simulink model "CP_ContrSys_Lin_b_n9945008"  (R2018b)
settings: Solver=VariableStepAuto  StartTime=0.0  StopTime=5  RelTol=1e-3
values from neighbouring files (symbols this model uses):
  Ab = [ 0 ,          0           , 1 , 0 ... (first row only)    [CP_ContrSys_Lin_b_MainFile_n9945008.m]
  Bb = [0;0;1/Mc;1/(l*Mc)]    [CP_ContrSys_Lin_b_MainFile_n9945008.m]
  Cb = [1,0,0,0 ... (first row only)    [CP_ContrSys_Lin_b_MainFile_n9945008.m]
  Kb = place(Ab, Bb, [-3,-4,-5,-6])    [CP_ContrSys_Lin_b_MainFile_n9945008.m]
  Lb = place(Ab',Cb', [-63,-64,-65,-66])'    [CP_ContrSys_Lin_b_MainFile_n9945008.m]
  x0 = [0.2 200*pi/180 0 0]'    [CP_ContrSys_Lin_b_MainFile_n9945008.m]
  xbar = [0;pi;0;0]    [CP_ContrSys_Lin_b_MainFile_n9945008.m]
settings Model: Creator=n9945008  LastModifiedBy=cody

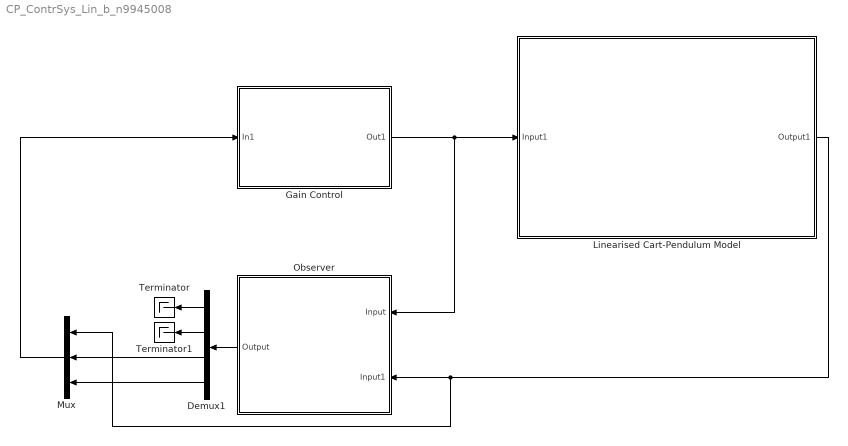
== system CP_ContrSys_Lin_b_n9945008 ==
  Demux1 : Demux
  Gain Control : Subsystem
  "Linearised Cart-Pendulum Model " : Subsystem
  Mux : Mux  Inputs=3
  Observer : Subsystem
  Terminator : Terminator
  Terminator1 : Terminator
  wires:
  Gain Control/1(Out1) -> "Linearised Cart-Pendulum Model "/1(Input1), Observer/1(Input)
  Observer/1(Output) -> Demux1/1
  Demux1/1 -> Terminator/1
  Demux1/2 -> Terminator1/1
  Demux1/3 -> Mux/2
  Demux1/4 -> Mux/3
  Mux/1 -> Gain Control/1(In1)
  "Linearised Cart-Pendulum Model "/1(Output1) -> Mux/1, Observer/2(Input1)

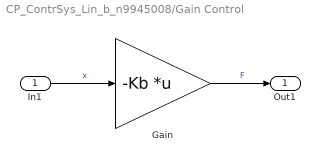
== system CP_ContrSys_Lin_b_n9945008/Gain Control ==
  In1 : Inport
  Gain : Gain  Gain=-Kb  Multiplication=Matrix(K*u)
  Out1 : Outport
  wires:
  In1/1 -> Gain/1  "x"
  Gain/1 -> Out1/1  "F"

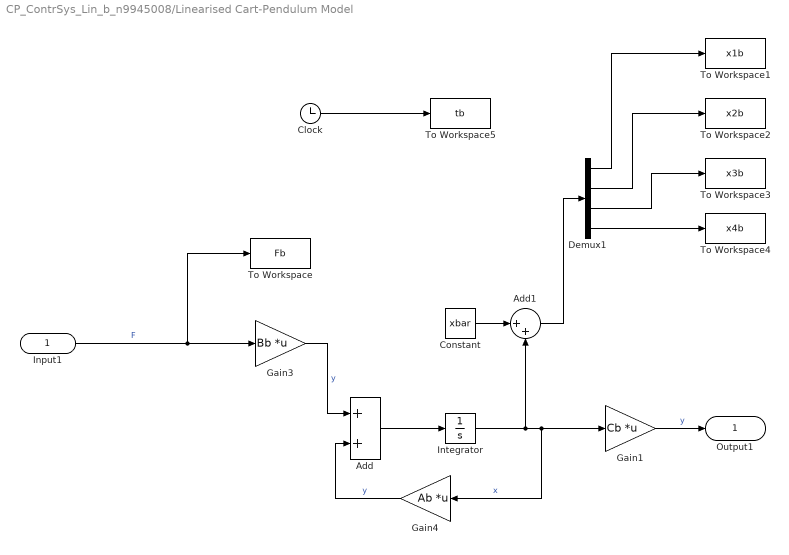
== system CP_ContrSys_Lin_b_n9945008/Linearised Cart-Pendulum Model  ==
  Input1 : Inport
  Add : Sum  Inputs=2
  Add1 : Sum  Inputs=|++
  Clock : Clock
  Constant : Constant  Value=xbar
  Demux1 : Demux
  Gain1 : Gain  Gain=Cb  Multiplication=Matrix(K*u)
  Gain3 : Gain  Gain=Bb  Multiplication=Matrix(K*u)
  Gain4 : Gain  Gain=Ab  Multiplication=Matrix(K*u)
  Integrator : Integrator  InitialCondition=x0-xbar
  To Workspace : ToWorkspace  VariableName=Fb  SampleTime=-1
      settings: Save2DSignal=2-D array (concatenate along first dimension)
  To Workspace1 : ToWorkspace  VariableName=x1b  SampleTime=-1
      settings: Save2DSignal=2-D array (concatenate along first dimension)
  To Workspace2 : ToWorkspace  VariableName=x2b  SampleTime=-1
      settings: Save2DSignal=2-D array (concatenate along first dimension)
  To Workspace3 : ToWorkspace  VariableName=x3b  SampleTime=-1
      settings: Save2DSignal=2-D array (concatenate along first dimension)
  To Workspace4 : ToWorkspace  VariableName=x4b  SampleTime=-1
      settings: Save2DSignal=2-D array (concatenate along first dimension)
  To Workspace5 : ToWorkspace  VariableName=tb  SampleTime=-1
      settings: Save2DSignal=2-D array (concatenate along first dimension)
  Output1 : Outport
  wires:
  Gain1/1 -> Output1/1  "y"
  Add/1 -> Integrator/1
  Demux1/3 -> To Workspace3/1
  Integrator/1 -> Gain1/1, Gain4/1, Add1/2  "x"
  Demux1/2 -> To Workspace2/1
  Clock/1 -> To Workspace5/1
  Gain3/1 -> Add/1  "y"
  Gain4/1 -> Add/2  "y"
  Demux1/4 -> To Workspace4/1
  Input1/1 -> To Workspace/1, Gain3/1  "F"
  Demux1/1 -> To Workspace1/1
  Constant/1 -> Add1/1
  Add1/1 -> Demux1/1

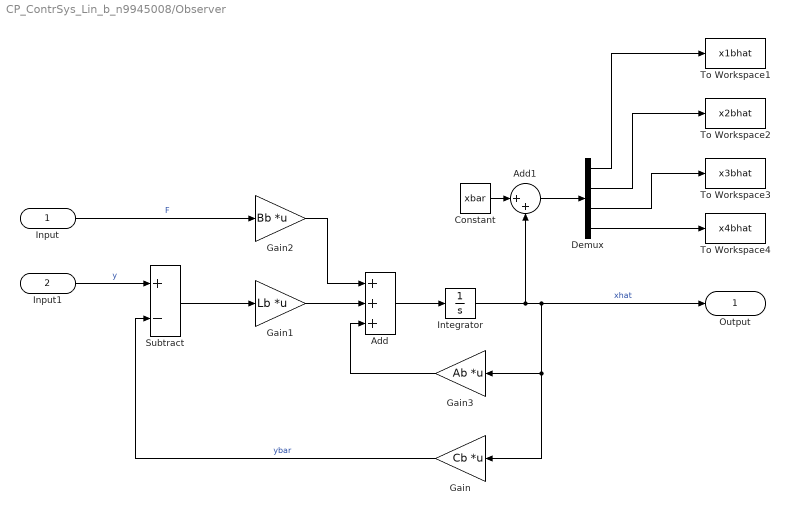
== system CP_ContrSys_Lin_b_n9945008/Observer ==
  Input : Inport
  Input1 : Inport  Port=2
  Add : Sum  Inputs=+++
  Add1 : Sum  Inputs=|++
  Constant : Constant  Value=xbar
  Demux : Demux
  Gain : Gain  Gain=Cb  Multiplication=Matrix(K*u)
  Gain1 : Gain  Gain=Lb  Multiplication=Matrix(K*u)
  Gain2 : Gain  Gain=Bb  Multiplication=Matrix(K*u)
  Gain3 : Gain  Gain=Ab  Multiplication=Matrix(K*u)
  Integrator : Integrator
  Subtract : Sum  Inputs=+-
  To Workspace1 : ToWorkspace  VariableName=x1bhat  SampleTime=-1
      settings: Save2DSignal=2-D array (concatenate along first dimension)
  To Workspace2 : ToWorkspace  VariableName=x2bhat  SampleTime=-1
      settings: Save2DSignal=2-D array (concatenate along first dimension)
  To Workspace3 : ToWorkspace  VariableName=x3bhat  SampleTime=-1
      settings: Save2DSignal=2-D array (concatenate along first dimension)
  To Workspace4 : ToWorkspace  VariableName=x4bhat  SampleTime=-1
      settings: Save2DSignal=2-D array (concatenate along first dimension)
  Output : Outport
  wires:
  Demux/1 -> To Workspace1/1
  Demux/4 -> To Workspace4/1
  Demux/2 -> To Workspace2/1
  Demux/3 -> To Workspace3/1
  Gain/1 -> Subtract/2  "ybar"
  Input1/1 -> Subtract/1  "y"
  Subtract/1 -> Gain1/1
  Gain1/1 -> Add/2
  Input/1 -> Gain2/1  "F"
  Gain2/1 -> Add/1
  Add/1 -> Integrator/1
  Gain3/1 -> Add/3
  Integrator/1 -> Output/1, Gain/1, Gain3/1, Add1/2  "xhat"
  Constant/1 -> Add1/1
  Add1/1 -> Demux/1
